simulink model "sensors"  (R2022b)
settings: Solver=VariableStepAuto  StartTime=0.0  StopTime=10.0  RelTol=1e-3
undefined symbols (not defined in the file or in its folder): filter_freq
libraries: simulink x1
settings Model: Creator=Tamer  LastModifiedBy=Andrey

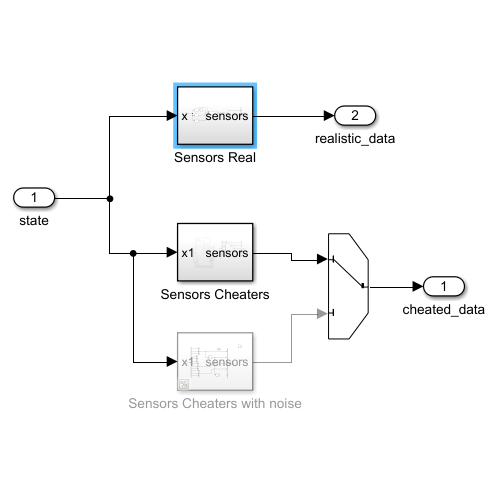
[thumbnail: Simulink's stored preview of the top-level diagram]
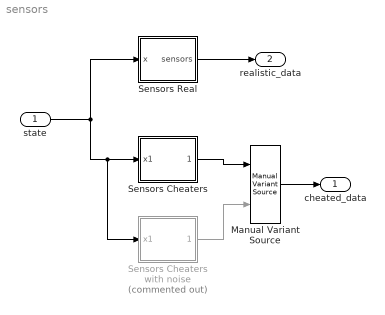
== system sensors ==
  state : Inport
  Manual Variant Source : simulink/Signal Routing/Manual Variant Source  NumChoices=2  LabelModeActiveChoice=V_1
  Sensors Cheaters : Subsystem
  Sensors Cheaters with noise : Subsystem  Commented=on
  Sensors Real : Subsystem
  cheated_data : Outport
  realistic_data : Outport  Port=2
  wires:
  state/1 -> Sensors Cheaters with noise/1(x1), Sensors Cheaters/1(x1), Sensors Real/1("x ")
  Sensors Real/1(sensors) -> realistic_data/1
  Sensors Cheaters/1(sensors) -> Manual Variant Source/1
  Sensors Cheaters with noise/1(sensors) -> Manual Variant Source/2
  Manual Variant Source/1 -> cheated_data/1

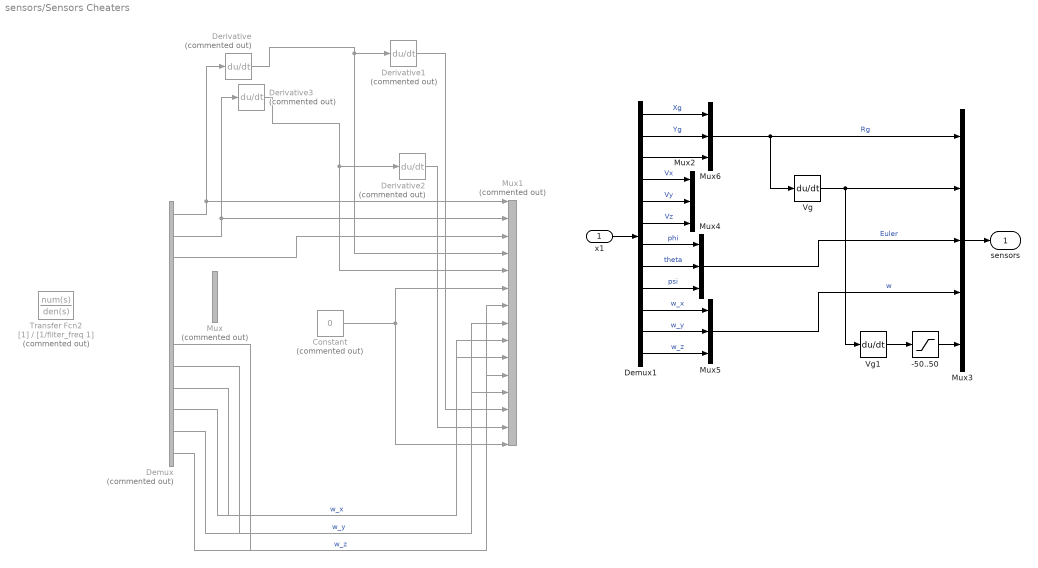
== system sensors/Sensors Cheaters ==
  x1 : Inport
  -50..50 : Saturate  UpperLimit=50  LowerLimit=-50
  Constant : Constant  Commented=on  Value=0
  Demux : Demux  Commented=on  Outputs=12
  Demux1 : Demux  Outputs=12
  Derivative{,1..3} (4 alike) : Derivative  Commented=on
  Mux : Mux  Commented=on  Inputs=3
  Mux1 : Mux  Commented=on  Inputs=15
  Mux{2,4..6} (4 alike) : Mux  Inputs=3
  Mux3 : Mux  Inputs=5
  Transfer Fcn2 : TransferFcn  Commented=on  Denominator=[1/filter_freq 1]
  Vg : Derivative
  Vg1 : Derivative
  sensors : Outport
  wires:
  Demux/3 -> Mux1/3
  Constant/1 -> Mux1/6, Mux1/15
  Demux/12 -> Mux1/11  "w_z"
  Demux/10 -> Mux1/10  "w_x"
  Demux/9 -> Mux1/9
  Demux/8 -> Mux1/8
  Demux/7 -> Mux1/7
  Demux/11 -> Mux1/12  "w_y"
  Demux/1 -> Mux1/1, Derivative/1
  Demux/2 -> Mux1/2, Derivative3/1
  Derivative/1 -> Derivative1/1, Mux1/4
  Derivative3/1 -> Derivative2/1, Mux1/5
  Derivative1/1 -> Mux1/13
  Derivative2/1 -> Mux1/14
  Demux1/12 -> Mux5/3  "w_z"
  Mux5/1 -> Mux3/4  "w"
  Mux4/1 -> Mux3/3  "Euler"
  Demux1/10 -> Mux5/1  "w_x"
  Demux1/8 -> Mux4/2  "theta"
  Demux1/7 -> Mux4/1  "phi"
  Demux1/6 -> Mux2/3  "Vz"
  Demux1/9 -> Mux4/3  "psi"
  Demux1/5 -> Mux2/2  "Vy"
  Demux1/4 -> Mux2/1  "Vx"
  Demux1/1 -> Mux6/1  "Xg"
  Demux1/2 -> Mux6/2  "Yg"
  Mux6/1 -> Vg/1, Mux3/1  "Rg"
  Vg/1 -> Mux3/2, Vg1/1
  Demux1/3 -> Mux6/3
  Mux3/1 -> sensors/1
  x1/1 -> Demux1/1
  Demux1/11 -> Mux5/2  "w_y"
  Vg1/1 -> -50..50/1
  -50..50/1 -> Mux3/5

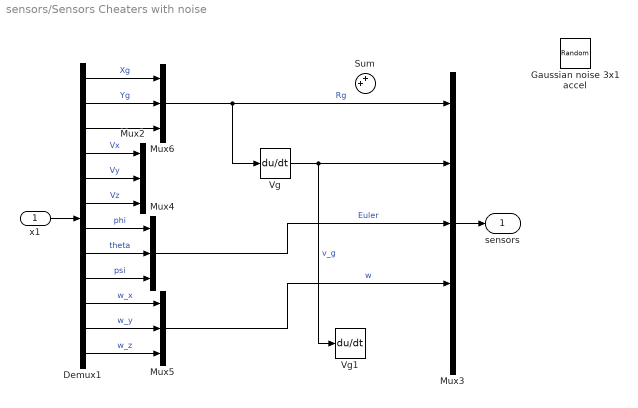
== system sensors/Sensors Cheaters with noise ==
  x1 : Inport
  Demux1 : Demux  Outputs=12
  Gaussian noise 3x1 accel : RandomNumber  Mean=[0 0 0]  Variance=[1 1 1] * 0.05  Seed=[23341 333 555]  SampleTime=0.005
  Mux{2,4..6} (4 alike) : Mux  Inputs=3
  Mux3 : Mux  Inputs=5
  Sum : Sum  Inputs=++|
  Vg : Derivative
  Vg1 : Derivative
  sensors : Outport
  wires:
  Demux1/12 -> Mux5/3  "w_z"
  Mux5/1 -> Mux3/4  "w"
  Mux4/1 -> Mux3/3  "Euler"
  Demux1/10 -> Mux5/1  "w_x"
  Demux1/8 -> Mux4/2  "theta"
  Demux1/7 -> Mux4/1  "phi"
  Demux1/6 -> Mux2/3  "Vz"
  Demux1/9 -> Mux4/3  "psi"
  Demux1/5 -> Mux2/2  "Vy"
  Demux1/4 -> Mux2/1  "Vx"
  Demux1/1 -> Mux6/1  "Xg"
  Demux1/2 -> Mux6/2  "Yg"
  Mux6/1 -> Vg/1, Mux3/1  "Rg"
  Vg/1 -> Mux3/2, Vg1/1  "v_g"
  Demux1/3 -> Mux6/3
  Mux3/1 -> sensors/1
  x1/1 -> Demux1/1
  Demux1/11 -> Mux5/2  "w_y"

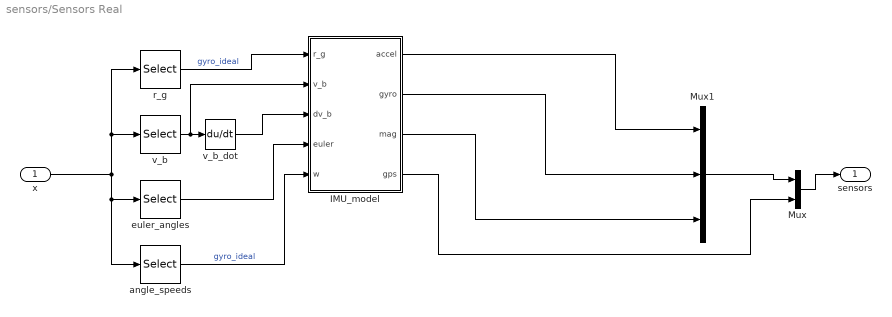
== system sensors/Sensors Real ==
  "x " : Inport
  IMU_model : Subsystem
  Mux : Mux  Inputs=2
  Mux1 : Mux  Inputs=3
  angle_speeds : Selector  InputPortWidth=12  IndexOptions=Index vector (dialog)  Indices=[10:12]  OutputSizes=1
  euler_angles : Selector  InputPortWidth=12  IndexOptions=Index vector (dialog)  Indices=[7:9]  OutputSizes=1
  r_g : Selector  InputPortWidth=12  IndexOptions=Index vector (dialog)  Indices=[1:3]  OutputSizes=1
  v_b : Selector  InputPortWidth=12  IndexOptions=Index vector (dialog)  Indices=[4:6]  OutputSizes=1
  v_b_dot : Derivative
  sensors : Outport
  wires:
  "x "/1 -> angle_speeds/1, euler_angles/1, r_g/1, v_b/1
  v_b_dot/1 -> IMU_model/3(dv_b)
  angle_speeds/1 -> IMU_model/5(w)  "gyro_ideal"
  v_b/1 -> IMU_model/2(v_b), v_b_dot/1
  euler_angles/1 -> IMU_model/4(euler)
  IMU_model/1(accel) -> Mux1/1
  IMU_model/2(gyro) -> Mux1/2
  r_g/1 -> IMU_model/1(r_g)  "gyro_ideal"
  IMU_model/3(mag) -> Mux1/3
  Mux1/1 -> Mux/1
  IMU_model/4(gps) -> Mux/2
  Mux/1 -> sensors/1

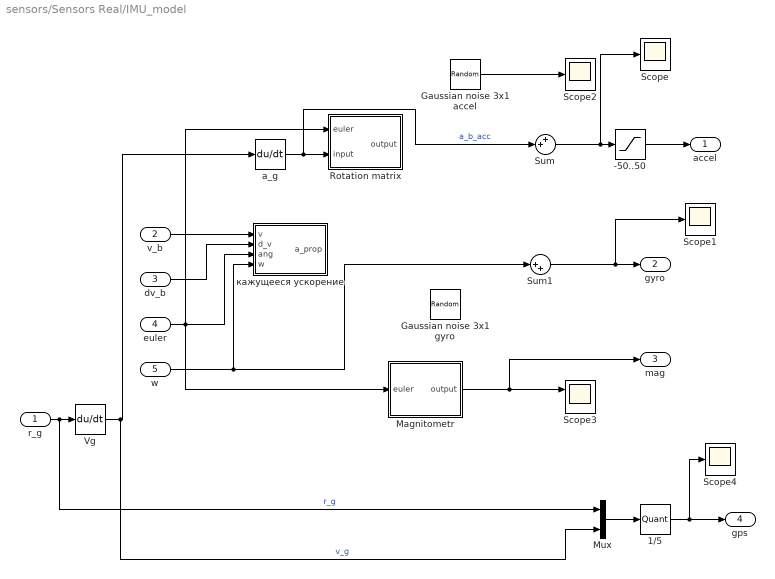
== system sensors/Sensors Real/IMU_model ==
  r_g : Inport
  v_b : Inport  Port=2
  dv_b : Inport  Port=3
  euler : Inport  Port=4
  w : Inport  Port=5
  -50..50 : Saturate  UpperLimit=50  LowerLimit=-50
  1/5 : Quantizer  QuantizationInterval=1/5
  Gaussian noise 3x1 accel : RandomNumber  Mean=[0 0 0]  Variance=[1 1 1] * 0.05  Seed=[23341 333 555]  SampleTime=0.005
  Gaussian noise 3x1 gyro : RandomNumber  Mean=[0 0 0]  Variance=[1 1 1] * deg2rad(0.1)  Seed=[23341 333 555]  SampleTime=0.005
  Magnitometr : MATLAB Function  TreatAsAtomicUnit=on
  Mux : Mux  Inputs=2
  Rotation matrix : MATLAB Function  TreatAsAtomicUnit=on
  Scope{,1..2,4} (4 alike) : Scope
  Scope3 : Scope  NumInputPorts=2
  Sum : Sum  Inputs=++|
  Sum1 : Sum  Inputs=|++
  Vg : Derivative
  a_g : Derivative
  кажущееся ускорение : MATLAB Function  TreatAsAtomicUnit=on
  accel : Outport
  gyro : Outport  Port=2
  mag : Outport  Port=3
  gps : Outport  Port=4  PortDimensions=[6 1]
  wires:
  v_b/1 -> кажущееся ускорение/1(v)
  dv_b/1 -> кажущееся ускорение/2(d_v)
  euler/1 -> кажущееся ускорение/3(ang), Magnitometr/1(euler), Rotation matrix/1(euler)
  w/1 -> Sum1/1, кажущееся ускорение/4(w)
  Gaussian noise 3x1 accel/1 -> Scope2/1
  Sum1/1 -> Scope1/1, gyro/1
  Sum/1 -> -50..50/1, Scope/1
  r_g/1 -> Mux/1, Vg/1  "r_g"
  -50..50/1 -> accel/1
  Magnitometr/1(output) -> mag/1, Scope3/1
  a_g/1 -> Sum/2, Rotation matrix/2(input)  "a_b_acc"
  Vg/1 -> Mux/2, a_g/1  "v_g"
  Mux/1 -> 1/5/1
  1/5/1 -> Scope4/1, gps/1

== matlab function sensors/Sensors Real/IMU_model/кажущееся ускорение ==
  data: v input; d_v input; ang input; a_prop output; w input
% Считает проекции кажущегося ускорения,
% эмуляция показателей акселерометра
% @v - скорость в связанной СК
% @d_v - производная скорости выше
% @ang - углы Эйлера
% @w - угловая скорость в проекциях на связанные оси
function a_prop = fcn(v, d_v, ang, w)
phi = ang(1);
theta = ang(2); 
g = 9.81;

% coriolis = [
%     w(3)*v(2) - w(2)*v(3);
%     w(1)*v(3) - w(3)*v(1);
%     w(2)*v(1) - w(1)*v(2)
% ];

coriolis = cross(v, w);

R = [
    sin(theta);
    cos(phi)*cos(theta);
    -sin(phi)*cos(theta)
];

a_prop = d_v - coriolis + R*g;

a_prop = d_v;

% a_prop(1) = d_v(1) - (w(3)*v(2) - w(2)*v(3)) + g*sin(theta);
% a_prop(2) = d_v(2) - (w(1)*v(3) - w(3)*v(1)) + g*cos(phi)*cos(theta);
% a_prop(3) = d_v(3) - (w(2)*v(1) - w(1)*v(2)) - g*sin(phi)*cos(theta);

== matlab function sensors/Sensors Real/IMU_model/Rotation matrix ==
  data: euler input; output output size=[3 1]; input input size=[3 1]
function output = fcn(euler, input)
phi = euler(1);
theta = euler(2);
psi = euler(3);

matrix = Utils.getRotationMatrix([phi theta psi]);
output = matrix * input; % в связанную

== matlab function sensors/Sensors Real/IMU_model/Magnitometr ==
  data: euler input; output output size=[3 1]
function output = fcn(euler)
phi = euler(1);
theta = euler(2);
psi = euler(3);

sumMagnetic = 40 * 1e-6;   % uT
mag_g = [1 0 0] * sumMagnetic;
mag_g = mag_g';
matrix = Utils.getRotationMatrix([phi theta psi]);  
output = matrix * mag_g;
